simulink model "exp5_7"  (Simulink 3.00)
settings: Solver=ode45  StartTime=0.0  StopTime=10.0  RelTol=1e-3

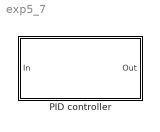
== system exp5_7 ==
  PID controller : Subsystem  mask(PID controller){kp=2, ki=3, kd=10}
      mask prompts: kp "比例系数kp"; ki "积分系数ki"; kd "微分系数kd"
      mask help:
      | 输入PID控制器的参数，比例系数、积分系数和微分系数
      | 表达式：
      | kp+ki/s+kd*s
      mask Help:
      | This block implements a PID controller where parameters are
      | entered for the Proportional,Integral and Derivative terms.
      mask Display: disp('PID')

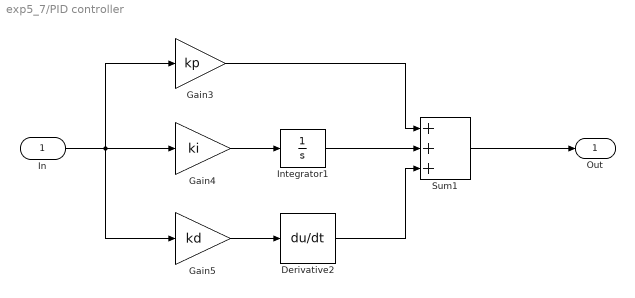
== system exp5_7/PID controller ==
  In : Inport  Port=1  PortWidth=-1  SampleTime=-1  DataType=auto
      settings: SignalType=auto
  Derivative2 : Derivative
  Gain3 : Gain  Gain=kp  SaturateOnIntegerOverflow=on
  Gain4 : Gain  Gain=ki  SaturateOnIntegerOverflow=on
  Gain5 : Gain  Gain=kd  SaturateOnIntegerOverflow=on
  Integrator1 : Integrator  ExternalReset=none  InitialConditionSource=internal  InitialCondition=0  LimitOutput=off  UpperSaturationLimit=inf  LowerSaturationLimit=-inf  ShowSaturationPort=off  ShowStatePort=off  AbsoluteTolerance=auto
  Sum1 : Sum  Inputs=+++  SaturateOnIntegerOverflow=on
  Out : Outport  Port=1
  wires:
  Gain4/1 -> Integrator1/1
  Gain5/1 -> Derivative2/1
  Gain3/1 -> Sum1/1
  Integrator1/1 -> Sum1/2
  Derivative2/1 -> Sum1/3
  Sum1/1 -> Out/1
  In/1 -> Gain4/1, Gain3/1, Gain5/1
